simulink model "WESDem_CalcState"  (R2016b)
settings: configuration reference "CodeGenConfigSet" (kept outside this file)
values from neighbouring files (symbols this model uses):
  WESDem_stCfg_C = Calibration.Parameter    [init_WESDem_CalcState.m]
  WESDem_stCfgvalid_C = Calibration.Parameter    [init_WESDem_CalcState.m]
  WESDem_stCrCtlInhibActv_C = Calibration.Parameter    [init_WESDem_CalcState.m]
  WESDem_stMode_C = Calibration.Parameter    [init_WESDem_CalcState.m]
  WESDem_stModevalid_C = Calibration.Parameter    [init_WESDem_CalcState.m]
  WESDem_swtEnaStrtModChng_C = Calibration.Parameter    [init_WESDem_CalcState.m]
  WESDem_tiBlockAftStrt_C = Calibration.Parameter    [init_WESDem_CalcState.m]
  WESDem_tiNeutr_C = Calibration.Parameter    [init_WESDem_CalcState.m]
  WESDem_trqThresNTC_C = Calibration.Parameter    [init_WESDem_CalcState.m]
  WESDem_vInhibCrCUI_C = Calibration.Parameter    [init_WESDem_CalcState.m]
  WESDem_vMaxAcc0_C = Calibration.Parameter    [init_WESDem_CalcState.m]
  WESDem_vMaxAcc1_C = Calibration.Parameter    [init_WESDem_CalcState.m]
  WESDem_vMaxAcc2_C = Calibration.Parameter    [init_WESDem_CalcState.m]
  WESDem_vMaxAcc3_C = Calibration.Parameter    [init_WESDem_CalcState.m]
undefined symbols (not defined in the file or in its folder): CrCUI_BttnState_conv, CruiseCtl_State_conv, EISGov_num_conv, EngState_conv, WESDem_CalcState_DT
libraries: simulink x50, CXLib x32
(part 2 of 2)

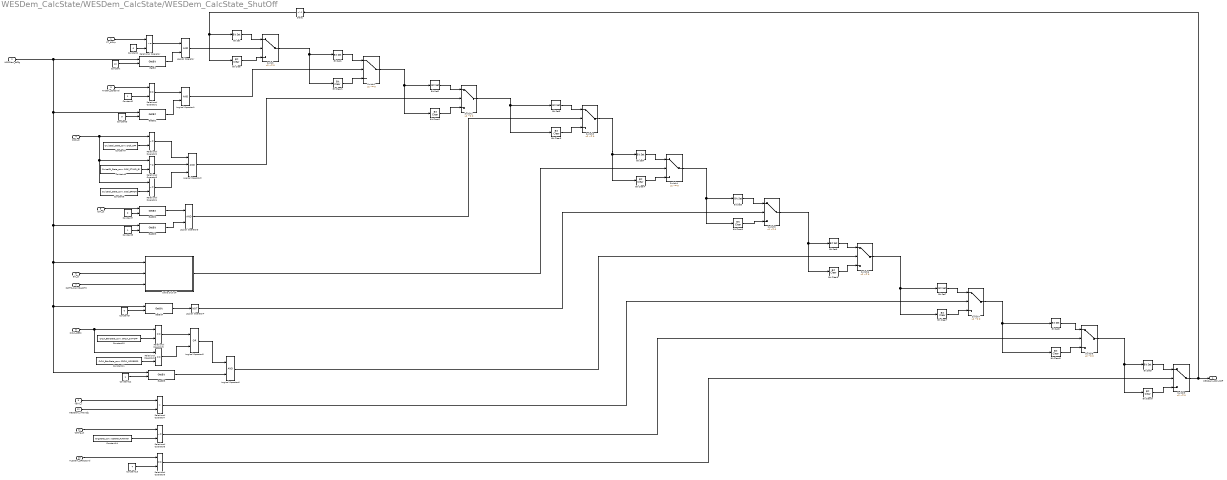
== system WESDem_CalcState/WESDem_CalcState/WESDem_CalcState_ShutOff ==
  PT_bGrip : Inport  Description=Grip is for sure present (the converter lockup clutch / the automated or manual clutch is completely closed and PT_bNoGrip = FALSE)  OutMin=0  OutMax=1  OutDataTypeStr=boolean
  WESDem_stCfg : Inport  Port=2  OutMin=0  OutMax=65535
  HndBrk_stDebVal : Inport  Description=Debounced value of Hand Brake switch  Port=3  OutMin=0  OutMax=255  OutDataTypeStr=State_uint8
  CrCtl_st : Inport  Description=Application parameter for Cruise Control state  Port=4
  Clth_st : Inport  Description=Clutch information  Port=5  OutMin=0  OutMax=255  OutDataTypeStr=State_uint8
  Brk_st : Inport  Description=Brake switch state  Port=6  OutMin=0  OutMax=255  OutDataTypeStr=State_uint8
  CoETS_trqInrDesNTC : Inport  Tag=Nm  Description=Additional desired engine friction Nm  Port=7  OutMin=-3276  OutMax=3276  OutDataTypeStr=Trq_Nm
  CrCUI_stBttn : Inport  Description=Application parameter for status button information  Port=8
  VehV_v : Inport  Tag=km/h  Description=Vehicle speed  Port=9  OutMin=0  OutMax=250  OutDataTypeStr=VehSpeed_km_h
  HLSDem_stReqCond : Inport  Description=Status of request for idle speed increase  Port=10  OutMin=0  OutMax=255  OutDataTypeStr=State_uint8
  CoEng_st : Inport  Description=Engine coordinator state  Port=11  OutDataTypeStr=Enum: EngState_conv
  WESDem_vMaxCfg : Inport  Description=Engine coordinator state  Port=12  OutDataTypeStr=VehSpeed_km_h
  Bit Clear : simulink/Logic and Bit Operations/Bit Clear  iBit=9
  Bit Clear1 : simulink/Logic and Bit Operations/Bit Clear  iBit=8
  Bit Clear2 : simulink/Logic and Bit Operations/Bit Clear  iBit=7
  Bit Clear3 : simulink/Logic and Bit Operations/Bit Clear  iBit=6
  Bit Clear4 : simulink/Logic and Bit Operations/Bit Clear  iBit=5
  Bit Clear5 : simulink/Logic and Bit Operations/Bit Clear  iBit=4
  Bit Clear6 : simulink/Logic and Bit Operations/Bit Clear  iBit=3
  Bit Clear7 : simulink/Logic and Bit Operations/Bit Clear  iBit=2
  Bit Clear8 : simulink/Logic and Bit Operations/Bit Clear  iBit=1
  Bit Clear9 : simulink/Logic and Bit Operations/Bit Clear  iBit=0
  Bit Set : simulink/Logic and Bit Operations/Bit Set  iBit=9
  Bit Set1 : simulink/Logic and Bit Operations/Bit Set  iBit=8
  Bit Set2 : simulink/Logic and Bit Operations/Bit Set  iBit=7
  Bit Set3 : simulink/Logic and Bit Operations/Bit Set  iBit=6
  Bit Set4 : simulink/Logic and Bit Operations/Bit Set  iBit=5
  Bit Set5 : simulink/Logic and Bit Operations/Bit Set  iBit=4
  Bit Set6 : simulink/Logic and Bit Operations/Bit Set  iBit=3
  Bit Set7 : simulink/Logic and Bit Operations/Bit Set  iBit=2
  Bit Set8 : simulink/Logic and Bit Operations/Bit Set  iBit=1
  Bit Set9 : simulink/Logic and Bit Operations/Bit Set  iBit=0
  Constant : Constant  Value=10  OutDataTypeStr=Inherit: Inherit via back propagation
  Constant1 : Constant  Value=0  OutDataTypeStr=Inherit: Inherit via back propagation
  Constant10 : Constant  Value=CrCUI_BttnState_conv.CRCUI_SWTOFF
  Constant11 : Constant  Value=CrCUI_BttnState_conv.CRCUI_MODEERR
  Constant12 : Constant  OutDataTypeStr=Inherit: Inherit via back propagation
  Constant13 : Constant  Value=4  OutDataTypeStr=Inherit: Inherit via back propagation
  Constant14 : Constant  Value=EngState_conv.COENG_RUNNING
  Constant2 : Constant  OutDataTypeStr=Inherit: Inherit via back propagation
  Constant3 : Constant  Value=9  OutDataTypeStr=Inherit: Inherit via back propagation
  Constant4 : Constant  Value=CruiseCtl_State_conv.CrCtl_OFF
  Constant5 : Constant  Value=CruiseCtl_State_conv.CrCtl_STAND_BY
  Constant6 : Constant  Value=CruiseCtl_State_conv.CrCtl_ERROR
  Constant7 : Constant  Value=0  OutDataTypeStr=Inherit: Inherit via back propagation
  Constant8 : Constant  Value=4  OutDataTypeStr=Inherit: Inherit via back propagation
  Constant9 : Constant  Value=0  OutDataTypeStr=Inherit: Inherit via back propagation
  Delay : Delay  DelayLength=1
  GetBit{,1,3..5} (5 alike) : CXLib/GetBit  dataTypeString=uint16  dataLength=0
      settings: AttributesFormatString=Get bit from %<dataTypeString>
  GetBit2 : CXLib/GetBit  dataTypeString=uint8  dataLength=0
      settings: AttributesFormatString=Get bit from %<dataTypeString>
  Logical Operator{,1,3,6} (4 alike) : Logic  AllPortsSameDT=off  OutDataTypeStr=boolean
  Logical Operator2 : Logic  Inputs=3  AllPortsSameDT=off  OutDataTypeStr=boolean
  Logical Operator4 : Logic  Operator=NOT  Inputs=1  AllPortsSameDT=off  OutDataTypeStr=boolean
  Logical Operator5 : Logic  Operator=OR  AllPortsSameDT=off  OutDataTypeStr=boolean
  Relational Operator{,2..4,8} (5 alike) : RelationalOperator  Operator=~=  OutDataTypeStr=boolean  RndMeth=Simplest
  Relational Operator{1,5..6,9} (4 alike) : RelationalOperator  Operator===  OutDataTypeStr=boolean  RndMeth=Simplest
  Relational Operator7 : RelationalOperator  Operator=>  OutDataTypeStr=boolean  RndMeth=Simplest
  Switch{,1..9} (10 alike) : Switch  Criteria=u2 ~= 0
  brake shut off : Subsystem
  WESDem_stShutOff : Outport  Description=Shut off conditions for the Working engine speed Demand  OutMin=0  OutMax=65535  OutDataTypeStr=State_uint16
  wires:
  CoETS_trqInrDesNTC/1 -> brake shut off/3(CoETS_trqInrDesNTC)
  Brk_st/1 -> brake shut off/2(Brk_st)
  Constant13/1 -> Relational Operator9/2
  Constant12/1 -> GetBit5/2
  Constant3/1 -> GetBit1/2
  Constant/1 -> GetBit/2
  Constant9/1 -> GetBit4/2
  Constant14/1 -> Relational Operator8/2
  GetBit5/1 -> Logical Operator6/2
  Relational Operator5/1 -> Logical Operator5/1
  Constant10/1 -> Relational Operator5/2
  GetBit4/1 -> Logical Operator4/1
  Relational Operator6/1 -> Logical Operator5/2
  HLSDem_stReqCond/1 -> Relational Operator9/1
  Logical Operator5/1 -> Logical Operator6/1
  CrCUI_stBttn/1 -> Relational Operator6/1, Relational Operator5/1
  Constant11/1 -> Relational Operator6/2
  VehV_v/1 -> Relational Operator7/1
  Constant8/1 -> GetBit3/2
  Relational Operator2/1 -> Logical Operator2/1
  Relational Operator4/1 -> Logical Operator2/3
  Clth_st/1 -> GetBit2/1
  Constant2/1 -> Relational Operator1/2
  Constant4/1 -> Relational Operator2/2
  Constant7/1 -> GetBit2/2
  GetBit3/1 -> Logical Operator3/2
  HndBrk_stDebVal/1 -> Relational Operator1/1
  Relational Operator1/1 -> Logical Operator1/1
  CrCtl_st/1 -> Relational Operator2/1, Relational Operator3/1, Relational Operator4/1
  Relational Operator3/1 -> Logical Operator2/2
  GetBit2/1 -> Logical Operator3/1
  GetBit1/1 -> Logical Operator1/2
  GetBit/1 -> Logical Operator/2
  Relational Operator/1 -> Logical Operator/1
  Constant5/1 -> Relational Operator3/2
  Constant6/1 -> Relational Operator4/2
  PT_bGrip/1 -> Relational Operator/1
  Constant1/1 -> Relational Operator/2
  WESDem_stCfg/1 -> GetBit5/1, GetBit4/1, brake shut off/1("WESDem_stCfg "), GetBit3/1, GetBit1/1, GetBit/1
  CoEng_st/1 -> Relational Operator8/1
  WESDem_vMaxCfg/1 -> Relational Operator7/2
  Switch9/1 -> Delay/1, WESDem_stShutOff/1
  Bit Clear/1 -> Switch/3
  Bit Set/1 -> Switch/1
  Logical Operator/1 -> Switch/2
  Switch/1 -> Bit Clear1/1, Bit Set1/1
  Bit Clear1/1 -> Switch1/3
  Bit Set1/1 -> Switch1/1
  Logical Operator1/1 -> Switch1/2
  Switch1/1 -> Bit Clear2/1, Bit Set2/1
  Bit Clear2/1 -> Switch2/3
  Bit Set2/1 -> Switch2/1
  Logical Operator2/1 -> Switch2/2
  Switch2/1 -> Bit Clear3/1, Bit Set3/1
  Bit Clear3/1 -> Switch3/3
  Bit Set3/1 -> Switch3/1
  Logical Operator3/1 -> Switch3/2
  Switch3/1 -> Bit Clear4/1, Bit Set4/1
  Bit Clear4/1 -> Switch4/3
  Bit Set4/1 -> Switch4/1
  brake shut off/1("WESDem_stShutOff.5 ") -> Switch4/2
  Switch4/1 -> Bit Clear5/1, Bit Set5/1
  Bit Clear5/1 -> Switch5/3
  Bit Set5/1 -> Switch5/1
  Logical Operator4/1 -> Switch5/2
  Bit Clear6/1 -> Switch6/3
  Bit Set6/1 -> Switch6/1
  Switch5/1 -> Bit Clear6/1, Bit Set6/1
  Logical Operator6/1 -> Switch6/2
  Switch6/1 -> Bit Clear7/1, Bit Set7/1
  Bit Clear7/1 -> Switch7/3
  Bit Set7/1 -> Switch7/1
  Relational Operator7/1 -> Switch7/2
  Switch7/1 -> Bit Clear8/1, Bit Set8/1
  Bit Clear8/1 -> Switch8/3
  Bit Set8/1 -> Switch8/1
  Switch8/1 -> Bit Clear9/1, Bit Set9/1
  Bit Clear9/1 -> Switch9/3
  Bit Set9/1 -> Switch9/1
  Relational Operator9/1 -> Switch9/2
  Relational Operator8/1 -> Switch8/2
  Delay/1 -> Bit Clear/1, Bit Set/1

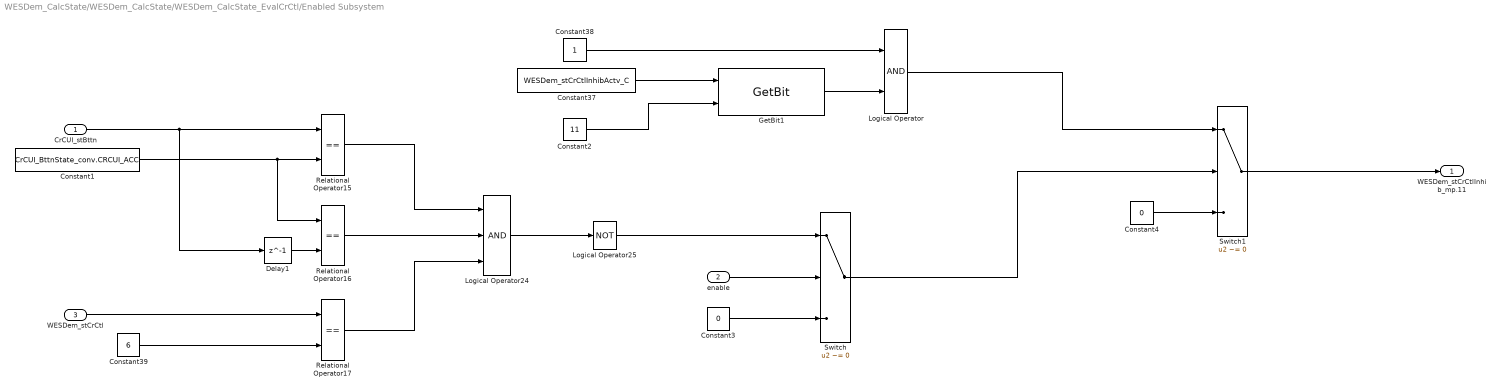
== system WESDem_CalcState/WESDem_CalcState/WESDem_CalcState_EvalCrCtl/Enabled Subsystem ==
  CrCUI_stBttn : Inport  Description=Application parameter for status button information
  enable : Inport  Port=2
  "WESDem_stCrCtl " : Inport  Description=Bit coded output message from engine stop function for low idle, egine shut off and crank control  Port=3  OutMin=0  OutMax=65535  OutDataTypeStr=uint16
  Constant1 : Constant  Value=CrCUI_BttnState_conv.CRCUI_ACC
  Constant2 : Constant  Value=11  OutDataTypeStr=Inherit: Inherit via back propagation
  Constant3 : Constant  Value=0  OutDataTypeStr=Inherit: Inherit via back propagation
  Constant37 : Constant  Value=WESDem_stCrCtlInhibActv_C
  Constant38 : Constant  OutDataTypeStr=Inherit: Inherit via back propagation
  Constant39 : Constant  Value=6  OutDataTypeStr=Inherit: Inherit via back propagation
  Constant4 : Constant  Value=0  OutDataTypeStr=Inherit: Inherit via back propagation
  Delay1 : Delay  DelayLength=1  InitialCondition=CrCUI_BttnState_conv.CRCUI_NEUTR
  GetBit1 : CXLib/GetBit  dataTypeString=uint16  dataLength=0
      settings: AttributesFormatString=Get bit from %<dataTypeString>
  Logical Operator : Logic  AllPortsSameDT=off  OutDataTypeStr=boolean
  Logical Operator24 : Logic  Inputs=3  AllPortsSameDT=off  OutDataTypeStr=boolean
  Logical Operator25 : Logic  Operator=NOT  AllPortsSameDT=off  OutDataTypeStr=boolean
  Relational Operator15 : RelationalOperator  Operator===  OutDataTypeStr=boolean  RndMeth=Simplest
  Relational Operator16 : RelationalOperator  Operator===  OutDataTypeStr=boolean  RndMeth=Simplest
  Relational Operator17 : RelationalOperator  Operator===  OutDataTypeStr=boolean  RndMeth=Simplest
  Switch : Switch  Criteria=u2 ~= 0  InputSameDT=on
  Switch1 : Switch  Criteria=u2 ~= 0  InputSameDT=on
  "WESDem_stCrCtlInhib_mp.11 " : Outport  Description=Operating mode change of the working engine speed demand  OutMin=0  OutMax=1  OutDataTypeStr=boolean
  wires:
  Constant1/1 -> Relational Operator16/1, Relational Operator15/2
  Delay1/1 -> Relational Operator16/2
  "WESDem_stCrCtl "/1 -> Relational Operator17/1
  Constant39/1 -> Relational Operator17/2
  Relational Operator16/1 -> Logical Operator24/2
  Relational Operator15/1 -> Logical Operator24/1
  Relational Operator17/1 -> Logical Operator24/3
  Logical Operator24/1 -> Logical Operator25/1
  CrCUI_stBttn/1 -> Delay1/1, Relational Operator15/1
  Logical Operator25/1 -> Switch/1
  Constant2/1 -> GetBit1/2
  Constant37/1 -> GetBit1/1
  GetBit1/1 -> Logical Operator/2
  Constant38/1 -> Logical Operator/1
  enable/1 -> Switch/2
  Constant3/1 -> Switch/3
  Switch/1 -> Switch1/2
  Logical Operator/1 -> Switch1/1
  Constant4/1 -> Switch1/3
  Switch1/1 -> "WESDem_stCrCtlInhib_mp.11 "/1

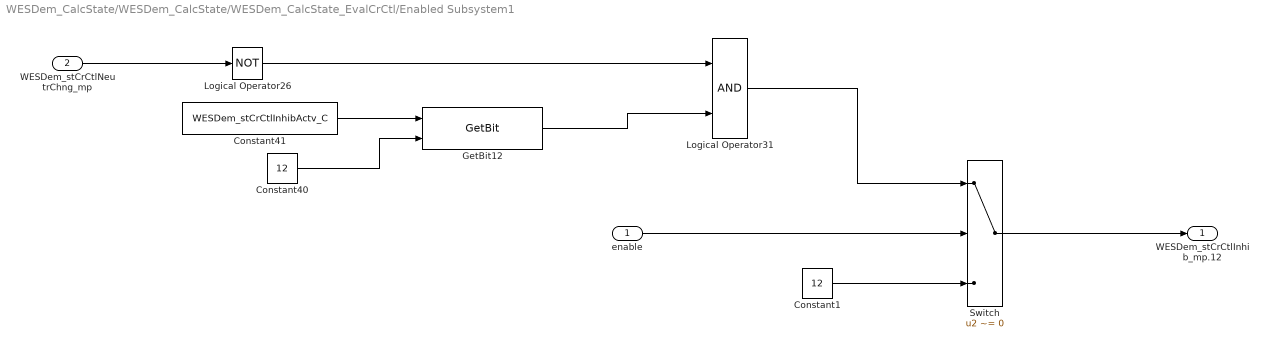
== system WESDem_CalcState/WESDem_CalcState/WESDem_CalcState_EvalCrCtl/Enabled Subsystem1 ==
  "enable " : Inport
  "WESDem_stCrCtlNeutrChng_mp " : Inport  Description=Brake switch state  Port=2  OutMin=0  OutMax=1  OutDataTypeStr=boolean
  Constant1 : Constant  Value=12  OutDataTypeStr=Inherit: Inherit via back propagation
  Constant40 : Constant  Value=12  OutDataTypeStr=Inherit: Inherit via back propagation
  Constant41 : Constant  Value=WESDem_stCrCtlInhibActv_C
  GetBit12 : CXLib/GetBit  dataTypeString=uint16  dataLength=0
      settings: AttributesFormatString=Get bit from %<dataTypeString>
  Logical Operator26 : Logic  Operator=NOT  AllPortsSameDT=off  OutDataTypeStr=boolean
  Logical Operator31 : Logic  AllPortsSameDT=off  OutDataTypeStr=boolean
  Switch : Switch  Criteria=u2 ~= 0  InputSameDT=on
  "WESDem_stCrCtlInhib_mp.12 " : Outport  Description=Operating mode change of the working engine speed demand  OutMin=0  OutMax=1  OutDataTypeStr=boolean
  wires:
  Constant41/1 -> GetBit12/1
  Constant40/1 -> GetBit12/2
  GetBit12/1 -> Logical Operator31/2
  "WESDem_stCrCtlNeutrChng_mp "/1 -> Logical Operator26/1
  Logical Operator26/1 -> Logical Operator31/1
  Logical Operator31/1 -> Switch/1
  "enable "/1 -> Switch/2
  Switch/1 -> "WESDem_stCrCtlInhib_mp.12 "/1
  Constant1/1 -> Switch/3

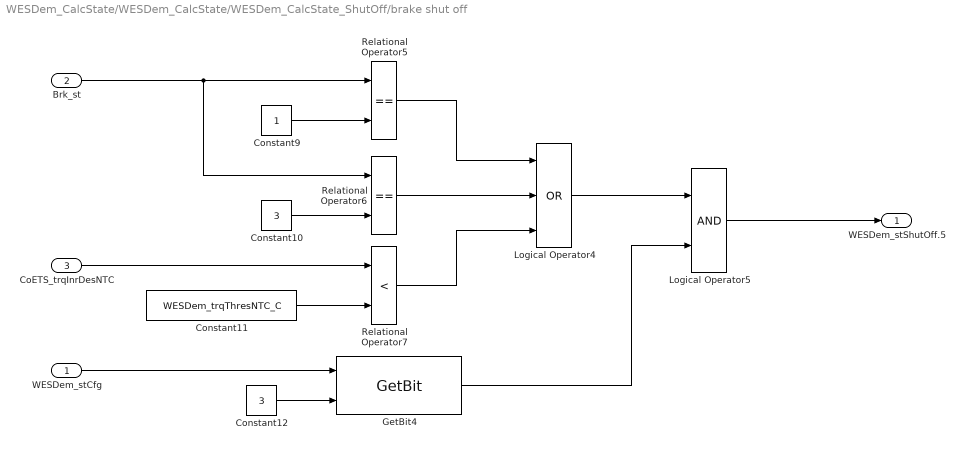
== system WESDem_CalcState/WESDem_CalcState/WESDem_CalcState_ShutOff/brake shut off ==
  "WESDem_stCfg " : Inport  Description=Application parameter for Cruise Control state  OutMin=0  OutMax=65535  OutDataTypeStr=State_uint16
  Brk_st : Inport  Description=Brake switch state  Port=2  OutMin=0  OutMax=255  OutDataTypeStr=State_uint8
  CoETS_trqInrDesNTC : Inport  Tag=Nm  Description=Additional desired engine friction Nm  Port=3  OutMin=-3276  OutMax=3276  OutDataTypeStr=Trq_Nm
  Constant10 : Constant  Value=3  OutDataTypeStr=Inherit: Inherit via back propagation
  Constant11 : Constant  Value=WESDem_trqThresNTC_C
  Constant12 : Constant  Value=3  OutDataTypeStr=Inherit: Inherit via back propagation
  Constant9 : Constant  OutDataTypeStr=Inherit: Inherit via back propagation
  GetBit4 : CXLib/GetBit  dataTypeString=uint16  dataLength=0
      settings: AttributesFormatString=Get bit from %<dataTypeString>
  Logical Operator4 : Logic  Operator=OR  Inputs=3  AllPortsSameDT=off  OutDataTypeStr=boolean
  Logical Operator5 : Logic  AllPortsSameDT=off  OutDataTypeStr=boolean
  Relational Operator5 : RelationalOperator  Operator===  OutDataTypeStr=boolean  RndMeth=Simplest
  Relational Operator6 : RelationalOperator  Operator===  OutDataTypeStr=boolean  RndMeth=Simplest
  Relational Operator7 : RelationalOperator  Operator=<  OutDataTypeStr=boolean  RndMeth=Simplest
  "WESDem_stShutOff.5 " : Outport  Description=Configuration of the actual operating mode  OutMin=0  OutMax=1  OutDataTypeStr=boolean
  wires:
  Relational Operator7/1 -> Logical Operator4/3
  Constant9/1 -> Relational Operator5/2
  CoETS_trqInrDesNTC/1 -> Relational Operator7/1
  Logical Operator4/1 -> Logical Operator5/1
  Constant10/1 -> Relational Operator6/2
  Relational Operator6/1 -> Logical Operator4/2
  Relational Operator5/1 -> Logical Operator4/1
  Constant12/1 -> GetBit4/2
  Brk_st/1 -> Relational Operator6/1, Relational Operator5/1
  GetBit4/1 -> Logical Operator5/2
  Constant11/1 -> Relational Operator7/2
  Logical Operator5/1 -> "WESDem_stShutOff.5 "/1
  "WESDem_stCfg "/1 -> GetBit4/1
